simulink model "testDeserialize"  (R2014a)
settings: Solver=FixedStepDiscrete  StartTime=0.0  StopTime=Inf  FixedStep=0.001  RelTol=1e-3
InitFcn:
  | testSerializedParams_Initialize();
undefined symbols (not defined in the file or in its folder): BusParam_TestBusOuter, TestBus_serializedParam
libraries: slrtlib x8
settings Model: BufferReuse=off  Creator=shenoylab  LastModifiedBy=shenoylab
settings SolverCC: EnableConcurrentExecution=on
settings DataIOCC: SignalLoggingSaveFormat=ModelDataLogs
settings OptimizationCC: BlockReduction=off  InlineParams=on  OptimizeBlockIOStorage=off  BufferReuse=off  GlobalBufferReuse=off  ExpressionFolding=off  LocalBlockOutputs=off
settings DebuggingCC: MultiTaskDSMMsg=warning  MultiTaskCondExecSysMsg=none  StateNameClashWarn=warning
settings HardwareCC: ProdIntDivRoundTo=Zero  ProdEndianess=LittleEndian  ProdHWDeviceType=Generic->32-bit x86 compatible
settings RTWCC: SystemTargetFile=slrt.tlc  TemplateMakefile=slrt_default_tmf  Description=Simulink Real-Time  GenerateReport=on  ProcessScript=slrt_make_rtw_hook  LaunchReport=on  IncludeERTFirstTime=on  RTWCompilerOptimization=On
settings CodeAppCC: MATLABSourceComments=on
settings SimulinkRealTimeCC: GeneratePreprocessorConditionals=Disable all  EnableShiftOperators=on

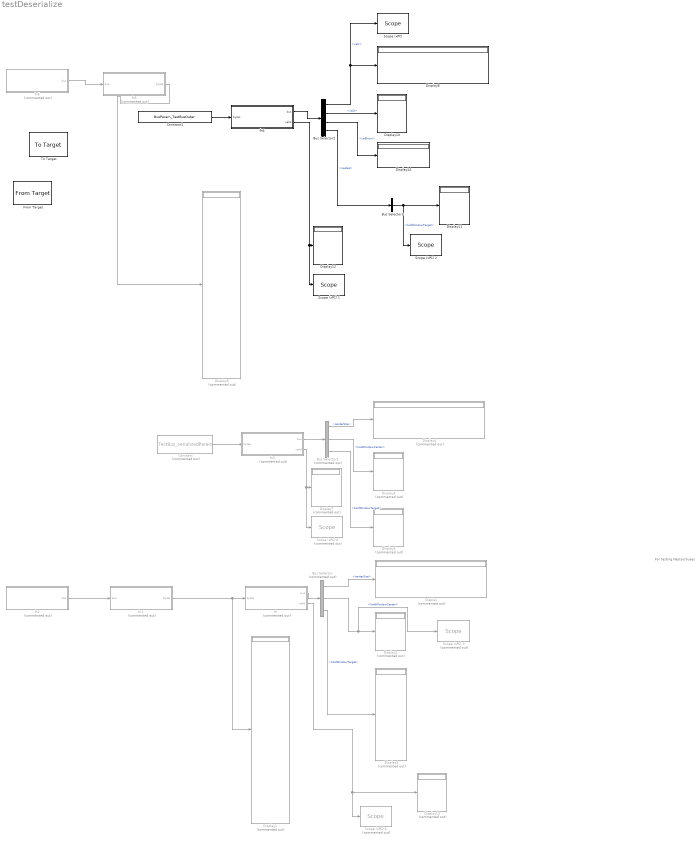
== system testDeserialize ==
  note: For testing Nested buses
  Bus Selector : BusSelector  Commented=on  OutputSignals=centerSize,holdWindowCenter,holdWindowTarget
  Bus Selector1 : BusSelector  Commented=on  OutputSignals=centerSize,holdWindowCenter,holdWindowTarget
  Bus Selector2 : BusSelector  OutputSignals=val1,val2,valEnum,nested
  Bus Selector3 : BusSelector  OutputSignals=holdWindowTarget
  Constant : Constant  Commented=on  Value=TestBus_serializedParam  OutDataTypeStr=uint8
  Constant1 : Constant  Value=BusParam_TestBusOuter  OutDataTypeStr=uint8
  Display{,1..7,9,13} (10 alike) : Display  Commented=on
  Display{8,10..12,14} (5 alike) : Display
  "From Target " : slrtlib/Displays and Logging/From Target   appname=''  blockpath=block  ts=1  isdefault=on
  "Scope (xPC) " : slrtlib/Displays and Logging/Scope   scopeno=1  scopetype=Target  autostart=on  viewmode=Numerical  formatstr='%15.6f'  grid=on  ylimits=[0,0]  nosamples=250  noprepostsamples=0  interleave=1  triggermode=FreeRun  triggersignal=1  trigsignalfromport=off  triggerlevel=0.0  triggerslope=Either  triggerscope=1  triggersample=0  filename=data.dat  mode=Lazy  writesize=512  autorestart=off  dynamicfilemode=off  maxwritefilesize=512*1024^2
  Scope (xPC) 1 : slrtlib/Displays and Logging/Scope   scopeno=2  scopetype=Target  autostart=on  viewmode=Numerical  formatstr='%15.6f'  grid=on  ylimits=[0,0]  nosamples=250  noprepostsamples=0  interleave=1  triggermode=FreeRun  triggersignal=1  trigsignalfromport=off  triggerlevel=0.0  triggerslope=Either  triggerscope=1  triggersample=0  filename=data.dat  mode=Lazy  writesize=512  autorestart=off  dynamicfilemode=off  maxwritefilesize=512*1024^2
  Scope (xPC) 2 : slrtlib/Displays and Logging/Scope   scopeno=3  scopetype=Target  autostart=on  viewmode=Numerical  formatstr='%15.6f'  grid=on  ylimits=[0,0]  nosamples=250  noprepostsamples=0  interleave=1  triggermode=FreeRun  triggersignal=1  trigsignalfromport=off  triggerlevel=0.0  triggerslope=Either  triggerscope=1  triggersample=0  filename=data.dat  mode=Lazy  writesize=512  autorestart=off  dynamicfilemode=off  maxwritefilesize=512*1024^2
  Scope (xPC) 3 : slrtlib/Displays and Logging/Scope   Commented=on  scopeno=4  scopetype=Target  autostart=on  viewmode=Numerical  formatstr='%15.6f'  grid=on  ylimits=[0,0]  nosamples=250  noprepostsamples=0  interleave=1  triggermode=FreeRun  triggersignal=1  trigsignalfromport=off  triggerlevel=0.0  triggerslope=Either  triggerscope=1  triggersample=0  filename=data.dat  mode=Lazy  writesize=512  autorestart=off  dynamicfilemode=off  maxwritefilesize=512*1024^2
  Scope (xPC) 4 : slrtlib/Displays and Logging/Scope   Commented=on  scopeno=5  scopetype=Target  autostart=on  viewmode=Numerical  formatstr='%15.6f'  grid=on  ylimits=[0,0]  nosamples=250  noprepostsamples=0  interleave=1  triggermode=FreeRun  triggersignal=1  trigsignalfromport=off  triggerlevel=0.0  triggerslope=Either  triggerscope=1  triggersample=0  filename=data.dat  mode=Lazy  writesize=512  autorestart=off  dynamicfilemode=off  maxwritefilesize=512*1024^2
  Scope (xPC) 6 : slrtlib/Displays and Logging/Scope   Commented=on  scopeno=6  scopetype=Target  autostart=on  viewmode=Numerical  formatstr='%15.6f'  grid=on  ylimits=[0,0]  nosamples=250  noprepostsamples=0  interleave=1  triggermode=FreeRun  triggersignal=1  trigsignalfromport=off  triggerlevel=0.0  triggerslope=Either  triggerscope=1  triggersample=0  filename=data.dat  mode=Lazy  writesize=512  autorestart=off  dynamicfilemode=off  maxwritefilesize=512*1024^2
  "To Target " : slrtlib/Displays and Logging/To Target   appname=''  blockpath=block  paramname=parameter  isdefault=on
  fn : MATLAB Function  Commented=on  TreatAsAtomicUnit=on
  fn1 : MATLAB Function  Commented=on  TreatAsAtomicUnit=on
  fn2 : MATLAB Function  Commented=on  TreatAsAtomicUnit=on
  fn3 : MATLAB Function  Commented=on  TreatAsAtomicUnit=on
  fn4 : MATLAB Function  TreatAsAtomicUnit=on
  fn5 : MATLAB Function  Commented=on  TreatAsAtomicUnit=on
  fn6 : MATLAB Function  Commented=on  TreatAsAtomicUnit=on
  wires:
  fn/1(bus) -> Bus Selector/1
  fn1/1(bytes) -> Display1/1, fn/1(bytes)
  fn2/1(bus) -> fn1/1(bus)
  Bus Selector/1 -> Display/1  "<centerSize>"
  Bus Selector/2 -> Scope (xPC) 3/1, Display2/1  "<holdWindowCenter>"
  Bus Selector/3 -> Display3/1  "<holdWindowTarget>"
  Constant/1 -> fn3/1(bytes)
  Bus Selector1/1 -> Display4/1  "<centerSize>"
  Bus Selector1/2 -> Display5/1  "<holdWindowCenter>"
  Bus Selector1/3 -> Display6/1  "<holdWindowTarget>"
  fn3/1(bus) -> Bus Selector1/1
  fn3/2(valid) -> Scope (xPC) 4/1, Display7/1
  Bus Selector2/1 -> "Scope (xPC) "/1, Display8/1  "<val1>"
  Bus Selector2/2 -> Display10/1  "<val2>"
  fn4/1(bus) -> Bus Selector2/1
  Bus Selector2/4 -> Bus Selector3/1  "<nested>"
  Bus Selector3/1 -> Scope (xPC) 2/1, Display11/1  "<holdWindowTarget>"
  fn4/2(valid) -> Scope (xPC) 1/1, Display12/1
  fn/2(valid) -> Scope (xPC) 6/1, Display13/1
  Bus Selector2/3 -> Display14/1  "<valEnum>"
  fn5/1(bytes) -> Display9/1
  fn6/1(bus) -> fn5/1(bus)
  Constant1/1 -> fn4/1(bytes)

== matlab function testDeserialize/fn1 ==
  data: bus input Bus: TestBus size=1; bytes output uint8 size=200
function bytes = serialize(bus)
%#codegen

bytes = testSerializedParamsLib.serializeBus_TestBus(bus);

== matlab function testDeserialize/fn ==
  data: bytes input uint8; bus output Bus: TestBus; valid output uint8 size=1
function [bus, valid] = deserialize(bytes)
%#codegen

[bus, valid] = testSerializedParamsLib.deserializeBus_TestBus(bytes);

== matlab function testDeserialize/fn2 ==
  data: bus output Bus: TestBus size=1
function bus = createBus()

coder.varsize('bus.centerSize', [3 3]);
coder.varsize('bus.holdWindowTarget', 30);
bus.centerSize = uint16([1 2; 3 4]);
bus.holdWindowCenter = uint8(15);
bus.holdWindowTarget = uint8('hello world')';

== matlab function testDeserialize/fn3 ==
  data: bytes input uint8; bus output Bus: TestBus; valid output uint8 size=1
function [bus, valid] = deserialize(bytes)
%#codegen

[bus, valid] = testSerializedParamsLib.deserializeBus_TestBus(bytes);

== matlab function testDeserialize/fn4 ==
  data: bytes input uint8; bus output Bus: TestBusOuter; valid output uint8 size=1
function [bus, valid] = deserialize(bytes)
%#codegen

[bus, valid] = testSerializedParamsLib.deserializeBus_TestBusOuter(bytes);

== matlab function testDeserialize/fn5 ==
  data: bus input Bus: TestBusOuter size=1; bytes output uint8 size=300
function bytes = serialize(bus)
%#codegen

bytes = testSerializedParamsLib.serializeBus_TestBusOuter(bus);

== matlab function testDeserialize/fn6 ==
  data: bus output Bus: TestBusOuter size=1
function bus = createBus()

bus = testSerializedParamsLib.initializeBus_TestBusOuter();
P1 = testSerializedParamsLib.initializeBus_TestBusInner();

P1.centerSize = uint8([1 2])';
P1.holdWindowCenter = uint8(2);
P1.holdWindowTarget = uint16(30);

bus.val1 = uint8(3);
bus.val2 = uint8('hello')';
bus.valEnum = TestEnum.eval3_longer;
bus.nested = P1;
